simulink model "MATE_PMSMDynamicSwitches"  (R2024b)
settings: Solver=FixedStepDiscrete  StartTime=0.0  StopTime=0.6  RelTol=1e-3  AbsTol=1e-3
PostLoadFcn:
  | Ts = 2e-6;
  | PMSMDynamicSwitches_init
InitFcn:
  | Ts = 2e-6;
  | PMSMDynamicSwitches_init
values from neighbouring files (symbols this model uses):
  J = 0.2    [PMSMDynamicSwitches_init.m]
  Tmax = 1.5*N*PM*Imax    (= 27)    [PMSMDynamicSwitches_init.m]
  Tsc = 1/fc    (= 5e-05)    [PMSMDynamicSwitches_init.m]
libraries: fl_lib x24, nesl_utility x19, simulink x3, ee_lib x3, batteryecm_lib x1, eePmsmFieldOrientedControl x1
(part 1 of 2)
Description:
  | Three-Phase PMSM Drive
settings Model: DataTypeOverride=Off  ModifiedByFormat=KD  Creator=Kyle Diller  LastModifiedBy=KD
settings SolverCC: AutoScaleAbsTol=off  MaxConsecutiveMinStep=2  ZeroCrossAlgorithm=Adaptive  AlgebraicLoopSolver=TrustRegion  MaxZcPerStep=1
settings DataIOCC: LimitDataPoints=on  MaxDataPoints=690000  SaveFormat=Array  ReturnWorkspaceOutputs=off  SignalLoggingName=logsout_ee_pmsm_drive
settings OptimizationCC: BlockReduction=off  ConditionallyExecuteInputs=off  DefaultParameterBehavior=Inlined  InheritOutputTypeSmallerThanSingle=on  ReuseModelBlockBuffer=off  LifeSpan=inf
settings DebuggingCC: AlgebraicLoopMsg=error  MaxConsecutiveZCsMsg=none  IgnoredZcDiagnostic=none  SingleTaskRateTransMsg=error  UnconnectedInputMsg=warning  UnconnectedOutputMsg=warning  UnconnectedLineMsg=warning  AllowSymbolicDim=off  PregeneratedLibrarySubsystemCodeDiagnostic=none  SFUnexpectedBacktrackingDiag=warning  SFNoUnconditionalDefaultTransitionDiag=warning  SFExecutionAtInitializationDiag=none  ArithmeticOperatorsInVariantConditions=warning
settings HardwareCC: ProdBitPerPointer=32  ProdBitPerSizeT=32  ProdBitPerPtrDiffT=32  ProdLargestAtomicFloat=None  ProdIntDivRoundTo=Undefined  ProdEndianess=Unspecified  ProdWordSize=32  ProdHWDeviceType=ASIC/FPGA->ASIC/FPGA  TargetBitPerPointer=64  TargetBitPerSizeT=64  TargetBitPerPtrDiffT=64  TargetLongLongMode=on  TargetIntDivRoundTo=Zero  TargetEndianess=LittleEndian  TargetWordSize=64  TargetHWDeviceType=Custom Processor->MATLAB Host Computer  ProdEqTarget=off
settings ModelReferenceCC: EnableRefExpFcnMdlSchedulingChecks=on  PropagateSignalLabelsOutOfModel=off
settings SFSimCC: SimUseLocalCustomCode=off
settings RTWCC: RTWUseLocalCustomCode=off  GPUComputeCapability=3.5  DLArmComputeVersion=19.05
settings CodeAppCC: StateflowObjectComments=on
settings GRTTargetCC: TargetLangStandard=C89/C90 (ANSI)
settings ConfigComp: CovMetricSettings=dw  CovSaveCumulativeToWorkspaceVar=on  CovSaveSingleToWorkspaceVar=on  CovExternalEMLEnable=off  CovSFcnEnable=off
settings SimscapeCC: SimscapeLogType=all  SimscapeLogSimulationStatistics=on  SimscapeLogName=simlog_ee_pmsm_drive  SimscapeLogDataHistory=690000

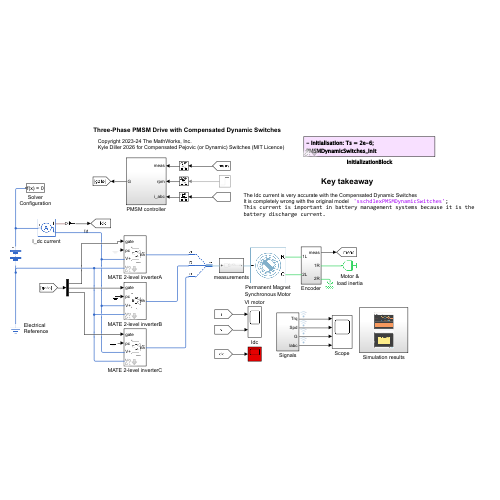
[thumbnail: Simulink's stored preview of the top-level diagram]
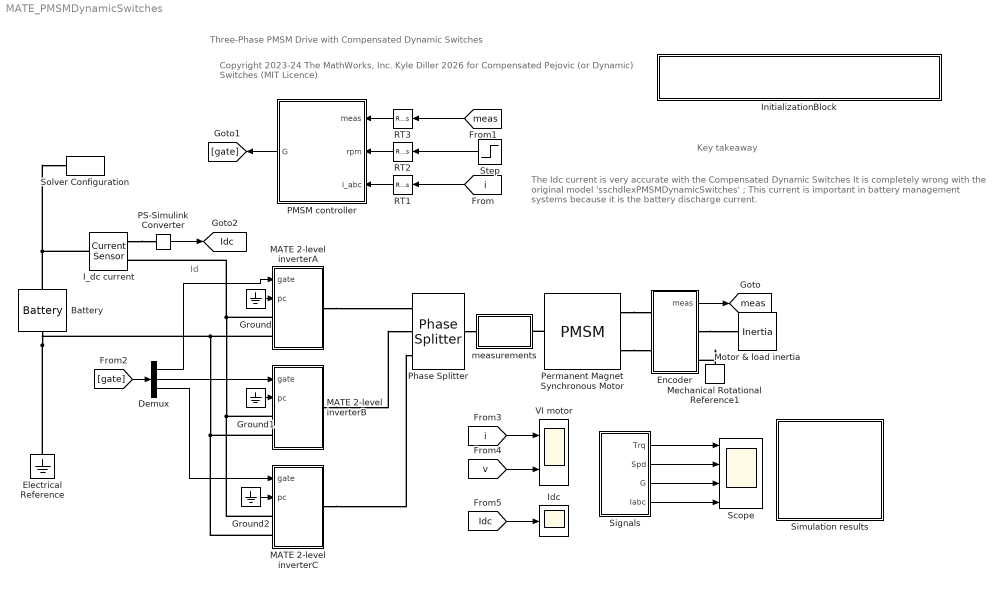
== system MATE_PMSMDynamicSwitches ==
  note: Key takeaway
  note: The Idc current is very accurate with the Compensated Dynamic Switches
      | It is completely wrong with the original model 'sschdlexPMSMDynamicSwitches' ;
      | This current is important in battery management systems because it is the battery discharge current.
  note: Id
  note: Three-Phase PMSM Drive with Compensated Dynamic Switches
  note: Copyright 2023-24 The MathWorks, Inc.
      | Kyle Diller 2026 for Compensated Pejovic (or Dynamic) Switches (MIT Licence)
  Battery : batteryecm_lib/Battery  Vnom=48 V  prm_dir=1  R1_dis=2 Ohm  R1_ch=2 Ohm  R1=0.001 Ohm  prm_AH=1  AH=14000 hr*A  V1=470 V  AH1=5000 hr*A  prm_R2=1  R2=inf Ohm  Tmeas=298.15 K  charge_measurement_port=simscape.enum.battery.enable.no  prm_dyn=1  Rp1=0.005 Ohm  tau1=30 s  Rp2=0.005 Ohm  tau2=30 s  Rp3=0.005 Ohm  tau3=30 s  Rp4=0.005 Ohm  tau4=30 s  Rp5=0.005 Ohm  tau5=30 s  prm_fade=1  N_fade=100  AH_fade=45 hr*A  R1_fade=2.02 Ohm  R1_ch_fade=2.02 Ohm  V1_fade=10.35 V  prm_age=1  prm_age_OCV=1  OCV_age=0.9  SOC_age=60  Tmeas_age=298.15 K  delta_time_age_vec=[0] d  temperature_age_vec=[273] K  OCV_scaling_age=2.2134e6  OCV_offset_age=1.632e6  temp_exp_age=0.515833569 V  t_exp_age=0.75  Vnom_T2=12 V  R1_T2=2.2 Ohm  R1_T2_dis=2.2 Ohm  R1_T2_ch=2.2 Ohm  V1_T2=11.4 V  R2_T2=2200 Ohm  Rp1_T2=0.005 Ohm  tau1_T2=30 s  Rp2_T2=0.005 Ohm  tau2_T2=30 s  Rp3_T2=0.005 Ohm  tau3_T2=30 s  Rp4_T2=0.005 Ohm  tau4_T2=30 s  Rp5_T2=0.005 Ohm  tau5_T2=30 s  Tmeas2=273.15 K  thermal_port=simscape.enum.thermaleffects.omit  thermal_mass=30000 J/K  i_specify=off  i_priority=None  i=0 A  i_nominal_specify=off  i_nominal_value=1  i_nominal_unit=A  v_specify=off  v_priority=None  v=0 V  v_nominal_specify=off  v_nominal_value=1  v_nominal_unit=V  charge_specify=on  charge_priority=High  charge=7000 hr*A  charge_nominal_specify=off  charge_nominal_value=1  charge_nominal_unit=A*hr  num_cycles_specify=off  num_cycles_priority=High  num_cycles=0  num_cycles_nominal_specify=off  num_cycles_nominal_value=1  num_cycles_nominal_unit=1  temperature_specify=off  temperature_priority=High  temperature=298.15 K  temperature_nominal_specify=off  temperature_nominal_value=1  temperature_nominal_unit=K
  Demux : Demux  Outputs=[2 2 2]
  Electrical Reference : fl_lib/Electrical/Electrical Elements/Electrical Reference
  Encoder : Subsystem
  Ground : Ground
  Ground1 : Ground
  Ground2 : Ground
  I_dc current : fl_lib/Electrical/Electrical Sensors/Current Sensor
  Idc : Scope
  InitializationBlock : Subsystem  AncestorBlock=simetranss/Usefulls/InitializationBlock  mask(Model Functions){InitVar=Ts = 2e-6;, InitFile=PMSMDynamicSwitches_init, prel=off, posl=on, inif=on}
      mask prompts: InitVar "Initialisation variables"; InitFile "Initialisation file (.m or .p)"; prel "Preload Function"; posl "PostLoad Function"; inif "InitFcn"
      mask init:
      | InitAll=[InitVar 10 InitFile];
      | if prel==1
      | 	set_param(bdroot, 'PreLoadFcn', InitAll);
      | else
      | 	set_param(bdroot, 'PreLoadFcn', '');
      | end
      | if inif==1
      | 	set_param(bdroot, 'InitFcn', InitAll);
      |     InitAll
      | else
      | 	set_param(bdroot, 'InitFcn', '');
      | end
      | 
      | if posl==1
      | 	set_param(bdroot, 'PostLoadFcn', InitAll);
      | else
      | 	set_param(bdroot, 'PostLoadFcn', '');
      | end
      | 
      | 
      | 
      | pos = get_param(gcb, 'Position');
      | width = pos(3) - pos(1); height = pos(4) - pos(2);
      mask DialogControl openfile Prompt: Open Initialisation file
      mask DialogControl openfile Callback:
      | ff1=get_param(gcb,'InitFile');
      | ff=replace(ff1,';','');
      | ff=replace(ff,'.m','');
      | ff=replace(ff,'.p','');
      | 
      | if ~isempty(strfind(ff1,'.p'))
      |     warning('p-file cannot be edited')
      | end
      | 
      | open(ff);
      mask Display:
      | text(5, height*0.5, [ ...
      |   ...
      | '- Initialisation: '  get_param(bdroot, 'InitFcn')  ...
      | ], ...
      | 'horizontalAlignment', 'left', 'verticalAlignment', 'middle') ;
  MATE 2-level inverterA : Subsystem  AncestorBlock=simetranss/FPGA/MATE 2-level inverter Pejovic  mask(MATE Compensated Pejovic 2-level inverter){Lon=1e-6, Ts=Ts}
      mask prompts: Lon "Conduction state inductance (H)"; Ts "Sample time (s)"
      mask help:
      | This block implements a 2-level IGBT/diode inverter with Pejovic switches.
      | The 2 switch are compensated at switching instant to transfer the L/C energy between the 2 switches, resulting in much better accuracy, much less spurious oscillation and power losses.
      |
      | The model supports dead-time on the gates. Internal logic makes the anti-parallel diode acts according to current direction when both gates are OFF.
      |
      | This model cannot interpolate or oversampled the gate action. Use of MATE 2-level inverter SWFHIZ is advised for this requirement.
      |
      | The 'pc' entry stands for 'precharge' when this input equals one and the upper gate level is one also, the upper switch acts as a simple resistance equal to the Pejovic resistance (L/h). In some converters, this property can be used to precharge the converter, as a pre-insersion resistance would do.
  MATE 2-level inverterB : Subsystem  AncestorBlock=simetranss/FPGA/MATE 2-level inverter Pejovic  mask(MATE Compensated Pejovic 2-level inverter){Lon=1e-6, Ts=Ts}
      mask prompts: Lon "Conduction state inductance (H)"; Ts "Sample time (s)"
      mask help:
      | This block implements a 2-level IGBT/diode inverter with Pejovic switches.
      | The 2 switch are compensated at switching instant to transfer the L/C energy between the 2 switches, resulting in much better accuracy, much less spurious oscillation and power losses.
      |
      | The model supports dead-time on the gates. Internal logic makes the anti-parallel diode acts according to current direction when both gates are OFF.
      |
      | This model cannot interpolate or oversampled the gate action. Use of MATE 2-level inverter SWFHIZ is advised for this requirement.
      |
      | The 'pc' entry stands for 'precharge' when this input equals one and the upper gate level is one also, the upper switch acts as a simple resistance equal to the Pejovic resistance (L/h). In some converters, this property can be used to precharge the converter, as a pre-insersion resistance would do.
  MATE 2-level inverterC : Subsystem  AncestorBlock=simetranss/FPGA/MATE 2-level inverter Pejovic  mask(MATE Compensated Pejovic 2-level inverter){Lon=1e-6, Ts=Ts}
      mask prompts: Lon "Conduction state inductance (H)"; Ts "Sample time (s)"
      mask help:
      | This block implements a 2-level IGBT/diode inverter with Pejovic switches.
      | The 2 switch are compensated at switching instant to transfer the L/C energy between the 2 switches, resulting in much better accuracy, much less spurious oscillation and power losses.
      |
      | The model supports dead-time on the gates. Internal logic makes the anti-parallel diode acts according to current direction when both gates are OFF.
      |
      | This model cannot interpolate or oversampled the gate action. Use of MATE 2-level inverter SWFHIZ is advised for this requirement.
      |
      | The 'pc' entry stands for 'precharge' when this input equals one and the upper gate level is one also, the upper switch acts as a simple resistance equal to the Pejovic resistance (L/h). In some converters, this property can be used to precharge the converter, as a pre-insersion resistance would do.
  Mechanical Rotational Reference1 : fl_lib/Mechanical/Rotational Elements/Mechanical Rotational Reference
  Motor & load inertia : fl_lib/Mechanical/Rotational Elements/Inertia  inertia=J kg*m^2  num_ports=foundation.enum.numPorts2.one  w_specify=on  w_priority=High  w=0 rpm  w_nominal_specify=off  w_nominal_value=1  w_nominal_unit=rad/s  t_specify=off  t_priority=High  t=0 N*m  t_nominal_specify=off  t_nominal_value=1  t_nominal_unit=N*m
  PMSM controller : Subsystem
  PS-Simulink Converter : nesl_utility/PS-Simulink Converter  PhysicalDomain=network_engine_domain  SubClassName=ps_output  LeftPortType=input  RightPortType=output  PseudoPeriodic=off  Frequencies=[]  VectorFormat=inherit  Unit=inherit  AffineConversion=off
  Permanent Magnet Synchronous Motor : ee_lib/Electromechanical/Permanent Magnet/PMSM  port_option=ee.enum.threePhasePort.composite  winding_type=ee.enum.statorconnection.wye  machine_param=ee.enum.pmsm.parameterization.constant  nPolePairs=N  pmflux_param=ee.enum.pmflux.fluxlinkage  pm_flux_linkage=PM Wb  torque_constant=0.18 N*m/A  back_emf_constant=0.18 V/(rad/s)  stator_param=ee.enum.statorparam.LdLqL0  Ld=Ld H  Lq=Lq H  idVec=[-200, 0, 200] A  iqVec=[-200, 0, 200] A  LdMatrix=0.0002 * ones(3, 3) H  LqMatrix=0.0002 * ones(3, 3) H  PmMatrix=0.1 * ones(3, 3) Wb  ktMatrix=0.18 * ones(3, 3) N*m/A  keMatrix=0.18 * ones(3, 3) V/(rad/s)  L0=L0 H  Ls=0.0002 H  Lm=0.00002 H  Ms=0.00002 H  Rs=Rs Ohm  zero_sequence=ee.enum.park.zerosequence.exclude  axes_param=ee.enum.rotorangle.qaxis  loss_param=ee.enum.ironloss.none  losses_oc=[0, 0, 0] W  losses_sc=[0, 0, 0] W  f_losses=60 Hz  Isc_losses=95 A  J=0 kg*m^2  lam=0 N*m/(rad/s)  i_d_specify=off  i_d_priority=None  i_d=0 A  i_d_nominal_specify=off  i_d_nominal_value=1  i_d_nominal_unit=A  i_q_specify=off  i_q_priority=None  i_q=0 A  i_q_nominal_specify=off  i_q_nominal_value=1  i_q_nominal_unit=A  torque_specify=off  torque_priority=None  torque=0 N*m  torque_nominal_specify=off  torque_nominal_value=1  torque_nominal_unit=N*m  angular_velocity_specify=on  angular_velocity_priority=None  angular_velocity=0 rpm  angular_velocity_nominal_specify=off  angular_velocity_nominal_value=1  angular_velocity_nominal_unit=rpm  angular_position_specify=on  angular_position_priority=High  angular_position=0 rad  angular_position_nominal_specify=off  angular_position_nominal_value=1  angular_position_nominal_unit=deg  alpha=3.93e-3 1/K  alpha_flux=-0.001 1/K  Tmeas=298.15 K  stator_thermal_mass=100 J/K  rotor_thermal_mass=200 J/K  Rm_percent_rotor=90  Rd_percent_rotor=30  temperatureA_specify=off  temperatureA_priority=High  temperatureA=25 degC  temperatureA_nominal_specify=off  temperatureA_nominal_value=1  temperatureA_nominal_unit=degC  temperatureB_specify=off  temperatureB_priority=High  temperatureB=25 degC  temperatureB_nominal_specify=off  temperatureB_nominal_value=1  temperatureB_nominal_unit=degC  temperatureC_specify=off  temperatureC_priority=High  temperatureC=25 degC  temperatureC_nominal_specify=off  temperatureC_nominal_value=1  temperatureC_nominal_unit=degC  temperatureR_specify=off  temperatureR_priority=High  temperatureR=25 degC  temperatureR_nominal_specify=off  temperatureR_nominal_value=1  temperatureR_nominal_unit=degC
      settings: InternalSimscapePortConfiguration="{\"Bottom\":[],\"Left\":[{\"id\":\"N\",\"label\":\"~\",\"type\":\"foundation.electrical.three_phase\"}],\"Right\":[{\"id\":\"R\",\"label\":\"R\",\"type\":\"foundation.mechanical.rotational.rotational\"},{\"id\":\"C\",\"label\":\"C\",\"type\":\"foundation.mechanical.rotational.rotational\"}],\"Top\":[]}"
  Phase Splitter : ee_lib/Connectors & References/Phase Splitter
  RT1 : RateTransition  OutPortSampleTime=Tsc
  RT2 : RateTransition  OutPortSampleTime=Tsc
  RT3 : RateTransition  OutPortSampleTime=Tsc
  Scope : Scope  NumInputPorts=4
  "Signals " : Subsystem
  Simulation results : Subsystem
  Solver Configuration : nesl_utility/Solver Configuration  PhysicalDomain=network_engine_domain  SubClassName=solver  LeftPortType=input  RightPortType=generic  Tones=[]  Harmonics=[]  SimulateNoise=off  Profile=off  UseLocalSampling=off  EnableSwitchedLinearOptims=on  FrequencyDomain=off  UseCCode=off  RelTol=0.001  AbsTol=1e-06  MinStep=1e-09  ToWorkspace=off  RevertToSquareIcSolve=off  NumHomotopyIterations=100  PhasorMode=off  PhasorModeNumHarmonics=1  ConsistencySolver=NEWTON_FTOL  IndexReductionMethod=DerivativeReplacement  DoDC=off  ResidualTolerance=1e-9  ConsistencyTolSource=GLOBAL  ConsistencyAbsTol=0.001  ConsistencyRelTol=0.001  ConsistencyTolFactor=0.001  UseLocalSolver=on  LocalSolverChoice=NE_PARTITIONING_ADVANCER  ResolveIndetEquations=on  FunctionEvalNumThread=1  LocalSolverSampleTime=Ts  DoFixedCost=on  MaxNonlinIter=4  MaxModeIter=2  ComputeImpulses=off  ImpulseIterations=2  LinearAlgebra=auto  LinearAlgebraNumThread=0  EquationFormulation=NE_TIME_EF  DelaysMemoryBudget=1024  AutomaticFiltering=on  FilteringTimeConstant=0.001  PartitionStorageMethod=AS_NEEDED  PartitionMemoryBudget=1024  PartitionMethod=FAST  MultibodyUseLocalSolver=off  MultibodyLocalSolverChoice=ODE1  MultibodyLocalSolverSampleTime=0.001
  Step : Step  Time=0.1  After=500  SampleTime=0
  VI motor : Scope  NumInputPorts=2
  measurements : Subsystem
  tag scope: Idc=global, meas=global
  wires:
  Step/1 -> RT2/1
  RT3/1 -> PMSM controller/1(meas)
  RT2/1 -> PMSM controller/2(rpm)
  RT1/1 -> PMSM controller/3(i_abc)
  "Signals "/2(Spd) -> Scope/2
  "Signals "/4(Iabc) -> Scope/4
  "Signals "/3(G) -> Scope/3
  "Signals "/1(Trq) -> Scope/1
  [i] -> RT1/1
  Encoder/1(meas) -> [meas]
  [meas] -> RT3/1
  PMSM controller/1(G) -> [gate]
  Demux/2 -> MATE 2-level inverterB/1(gate)
  Demux/1 -> MATE 2-level inverterA/1(gate)
  Demux/3 -> MATE 2-level inverterC/1(gate)
  [gate] -> Demux/1
  [i] -> VI motor/1
  [v] -> VI motor/2
  PS-Simulink Converter/1 -> [Idc]
  [Idc] -> Idc/1
  Ground/1 -> MATE 2-level inverterA/2(pc)
  Ground1/1 -> MATE 2-level inverterB/2(pc)
  Ground2/1 -> MATE 2-level inverterC/2(pc)
  connections:
  Battery/LConn1 -- I_dc current/LConn1 -- Solver Configuration/RConn1
  Permanent Magnet Synchronous Motor/RConn1 -- Encoder/LConn1
  Permanent Magnet Synchronous Motor/RConn2 -- Encoder/LConn2
  Encoder/RConn1 -- Motor & load inertia/LConn1
  Mechanical Rotational Reference1/LConn1 -- Encoder/RConn2
  Electrical Reference/LConn1 -- MATE 2-level inverterA/LConn2 -- MATE 2-level inverterC/LConn2 -- MATE 2-level inverterB/LConn2 -- Battery/RConn1
  I_dc current/RConn1 -- PS-Simulink Converter/LConn1
  MATE 2-level inverterA/LConn1 -- I_dc current/RConn2 -- MATE 2-level inverterC/LConn1 -- MATE 2-level inverterB/LConn1
  MATE 2-level inverterA/RConn1 -- Phase Splitter/RConn1
  MATE 2-level inverterB/RConn1 -- Phase Splitter/RConn2
  MATE 2-level inverterC/RConn1 -- Phase Splitter/RConn3
  Phase Splitter/LConn1 -- measurements/LConn1
  Permanent Magnet Synchronous Motor/LConn1 -- measurements/RConn1

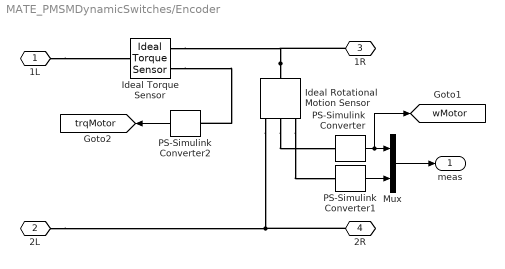
== system MATE_PMSMDynamicSwitches/Encoder ==
  Ideal Rotational Motion Sensor : fl_lib/Mechanical/Mechanical Sensors/Ideal Rotational Motion Sensor  reference=foundation.enum.MeasurementReference.difference  acceleration_port=false  velocity_port=true  position_port=true  wrap_angle=simscape.enum.onoff.off  offset=0 deg
  Ideal Torque Sensor : fl_lib/Mechanical/Mechanical Sensors/Ideal Torque Sensor
  Mux : Mux  Inputs=2
  PS-Simulink Converter : nesl_utility/PS-Simulink Converter  PhysicalDomain=network_engine_domain  SubClassName=ps_output  LeftPortType=input  RightPortType=output  PseudoPeriodic=off  Frequencies=[]  VectorFormat=1-D array  Unit=rad/s  AffineConversion=off
  PS-Simulink Converter1 : nesl_utility/PS-Simulink Converter  PhysicalDomain=network_engine_domain  SubClassName=ps_output  LeftPortType=input  RightPortType=output  PseudoPeriodic=off  Frequencies=[]  VectorFormat=1-D array  Unit=rad  AffineConversion=off
  PS-Simulink Converter2 : nesl_utility/PS-Simulink Converter  PhysicalDomain=network_engine_domain  SubClassName=ps_output  LeftPortType=input  RightPortType=output  PseudoPeriodic=off  Frequencies=[]  VectorFormat=1-D array  Unit=N*m  AffineConversion=off
  1L : PMIOPort  Side=Left
  2L : PMIOPort  Port=2  Side=Left
  1R : PMIOPort  Port=3  Side=Right
  2R : PMIOPort  Port=4  Side=Right
  meas : Outport  VectorParamsAs1DForOutWhenUnconnected=off
  tag scope: trqMotor=global, wMotor=global
  wires:
  PS-Simulink Converter2/1 -> [trqMotor]
  Mux/1 -> meas/1
  PS-Simulink Converter1/1 -> Mux/2
  PS-Simulink Converter/1 -> [wMotor], Mux/1
  connections:
  Ideal Torque Sensor/RConn2 -- PS-Simulink Converter2/LConn1
  1L/RConn1 -- Ideal Torque Sensor/LConn1
  2R/RConn1 -- 2L/RConn1 -- Ideal Rotational Motion Sensor/RConn1
  Ideal Rotational Motion Sensor/LConn1 -- 1R/RConn1 -- Ideal Torque Sensor/RConn1
  Ideal Rotational Motion Sensor/RConn2 -- PS-Simulink Converter/LConn1
  Ideal Rotational Motion Sensor/RConn3 -- PS-Simulink Converter1/LConn1

== system MATE_PMSMDynamicSwitches/InitializationBlock ==

== system MATE_PMSMDynamicSwitches/MATE 2-level inverterA ==
  gate : Inport
  pc : Inport  Port=2
  Add : Sum  Inputs=-+
  Demux2 : Demux  Outputs=2
  IGBT/Diode logic : Subsystem
  Unit Delay2 : UnitDelay  SampleTime=Ts  HasFrameUpgradeWarning=on
  lower : Subsystem  AncestorBlock=simetranss/FPGA/Pejovic L-C-switch component  mask(Pejovic Element for FPGA simulation){typ=2-level inverter switch, Lon=Lon, L=1, C=1, otherSW='coming soon', Ts=Ts, pcbp=off}
      mask prompts: typ "Element type"; Lon "Switch equivalent ON inductance (H)"; L "Inductor inductance (H)"; C "Capacitor capacitance (F)"; otherSW "Linked Compensated switch name"; Ts "Sample Time (s)"; pcbp "Precharge bypass (inverter only)"
      mask help:
      | Pejovic L-C-Switch element  in SimScape
      |
      | Implements either  an inductor, a capacitor or a switch using the Pejovic constant admittance method.
      |
      | For the Switch option, the user only has to select the equivalent ON-state inductance of the model, the corresponding Capacitance is computed internally. In the Pejovic model, Ts/Lon=Coff/Ts (Backward Euler) resulting in a constant admittance for the DAE solver.
      |
      |
      | Input signals;
      |
      | gate: the switch gate value (1 for ON , 0 for OFF) (with Switch option)
      mask init:
      | block=gcb;
      | Xcomp=0;
      | 
      | typp=get_param(block,'typ');
      | bp=get_param(block,'pcbp');
      | if isequal(typp,'Switch')
      |     replace_block (block ,'Followlinks' ,'on' ,'Name' ,'gate' ,'BlockType' ,'Constant' ,'Inport' ,'noprompt' ); 
      |     replace_block (block ,'Followlinks' ,'on' ,'Name' ,'init_in' ,'BlockType' ,'Inport' ,'Constant' ,'noprompt'  );
      |     replace_block (block ,'Followlinks' ,'on' ,'Name' ,'init_out' ,'BlockType' ,'Outport' ,'Terminator' ,'noprompt'  );
      |     Rsw=Lon/Ts;
      |     txt='Switch';
      | 
      | elseif isequal(typp,'Inductor')
      |     replace_block (block ,'Followlinks' ,'on' ,'Name' ,'gate' ,'BlockType' ,'Inport' ,'Constant' ,'noprompt' ); 
      |     set_param([block '/gate'],'Value','1');
      |     replace_block (block ,'Followlinks' ,'on' ,'Name' ,'init_in' ,'BlockType' ,'Inport' ,'Constant' ,'noprompt'  ); 
      |     replace_block (block ,'Followlinks' ,'on' ,'Name' ,'init_out' ,'BlockType' ,'Outport' ,'Terminator' ,'noprompt'  );
      |     Rsw=L/Ts;
      |     txt='L';
      | elseif isequal(typp,'Capacitor')
      |     replace_block (block ,'Followlinks' ,'on' ,'Name' ,'gate' ,'BlockType' ,'Inport' ,'Constant' ,'noprompt' ); 
      |     set_param([block '/gate'],'Value','0');
      |     replace_block (block ,'Followlinks' ,'on' ,'Name' ,'init_in' ,'BlockType' ,'Inport' ,'Constant' ,'noprompt'  );
      |     replace_block (block ,'Followlinks' ,'on' ,'Name' ,'init_out' ,'BlockType' ,'Outport' ,'Terminator' ,'noprompt'  );
      |     Rsw=Ts/C;
      |     txt='C';
      | elseif isequal(typp,'2-level inverter switch')
      |     replace_block (block ,'Followlinks' ,'on' ,'Name' ,'gate' ,'BlockType' ,'Constant' ,'Inport' ,'noprompt' ); 
      |     replace_block (block ,'Followlinks' ,'on' ,'Name' ,'init_in' ,'BlockType' ,'Constant' ,'Inport','noprompt'  );
      |     replace_block (block ,'Followlinks' ,'on' ,'Name' ,'init_out' ,'BlockType' ,'Terminator' ,'Outport' ,'noprompt'  );
      |     Rsw=Lon/Ts;
      |     txt='Inverter half';
      |     Xcomp=1;
      | 
      | else
      | end
      | 
      | if isequal(typp,'2-level inverter switch')  && isequal(bp,'on')
      |         replace_block (block ,'Followlinks' ,'on' ,'Name' ,'Bypass' ,'BlockType' ,'Ground' ,'Inport' ,'noprompt' ); 
      | else
      |         replace_block (block ,'Followlinks' ,'on' ,'Name' ,'Bypass' ,'BlockType' ,'Inport' ,'Ground' ,'noprompt' ); 
      | end
      | 
      | 
      | 
      | 
      | if Ts>2e-6
      |     %warndlg(['Sample Time of ' num2str(Ts) ' s. may be somehow large for the Pejovic switch to be accurate. Sample time below 2 us are recommended.'])
      | end
      mask TypeOptions typ: Switch | Inductor | Capacitor | 2-level inverter switch
      mask Display: disp(txt)
  upper : Subsystem  AncestorBlock=simetranss/FPGA/Pejovic L-C-switch component  mask(Pejovic Element for FPGA simulation){typ=2-level inverter switch, Lon=Lon, L=1, C=1, otherSW='coming soon', Ts=Ts, pcbp=on}
      mask prompts: typ "Element type"; Lon "Switch equivalent ON inductance (H)"; L "Inductor inductance (H)"; C "Capacitor capacitance (F)"; otherSW "Linked Compensated switch name"; Ts "Sample Time (s)"; pcbp "Precharge bypass (inverter only)"
      mask help:
      | Pejovic L-C-Switch element  in SimScape
      |
      | Implements either  an inductor, a capacitor or a switch using the Pejovic constant admittance method.
      |
      | For the Switch option, the user only has to select the equivalent ON-state inductance of the model, the corresponding Capacitance is computed internally. In the Pejovic model, Ts/Lon=Coff/Ts (Backward Euler) resulting in a constant admittance for the DAE solver.
      |
      |
      | Input signals;
      |
      | gate: the switch gate value (1 for ON , 0 for OFF) (with Switch option)
      mask init: same as MATE_PMSMDynamicSwitches/MATE 2-level inverterA/lower
      mask TypeOptions typ: Switch | Inductor | Capacitor | 2-level inverter switch
      mask Display: disp(txt)
  V+ : PMIOPort  Side=Left
  Va : PMIOPort  Port=2  Side=Right
  V- : PMIOPort  Port=3  Side=Left
  wires:
  pc/1 -> upper/3(Bypass)
  lower/1(init_out) -> upper/2(init_in)
  upper/1(init_out) -> lower/2(init_in)
  Demux2/1 -> upper/1(gate)
  Demux2/2 -> lower/1(gate)
  [iout] -> IGBT/Diode logic/2(u)
  gate/1 -> IGBT/Diode logic/1(In1)
  IGBT/Diode logic/1(UpperLower) -> Demux2/1
  Add/1 -> Unit Delay2/1
  Unit Delay2/1 -> [iout]
  upper/2(iout) -> Add/1
  lower/2(iout) -> Add/2
  connections:
  lower/RConn1 -- V-/RConn1
  upper/LConn1 -- V+/RConn1
  lower/LConn1 -- Va/RConn1 -- upper/RConn1

== system MATE_PMSMDynamicSwitches/MATE 2-level inverterB ==
  gate : Inport
  pc : Inport  Port=2
  Add : Sum  Inputs=-+
  Demux2 : Demux  Outputs=2
  IGBT/Diode logic : Subsystem
  Unit Delay2 : UnitDelay  SampleTime=Ts  HasFrameUpgradeWarning=on
  lower : Subsystem  AncestorBlock=simetranss/FPGA/Pejovic L-C-switch component  mask(Pejovic Element for FPGA simulation){typ=2-level inverter switch, Lon=Lon, L=1, C=1, otherSW='coming soon', Ts=Ts, pcbp=off}
      mask prompts: typ "Element type"; Lon "Switch equivalent ON inductance (H)"; L "Inductor inductance (H)"; C "Capacitor capacitance (F)"; otherSW "Linked Compensated switch name"; Ts "Sample Time (s)"; pcbp "Precharge bypass (inverter only)"
      mask help:
      | Pejovic L-C-Switch element  in SimScape
      |
      | Implements either  an inductor, a capacitor or a switch using the Pejovic constant admittance method.
      |
      | For the Switch option, the user only has to select the equivalent ON-state inductance of the model, the corresponding Capacitance is computed internally. In the Pejovic model, Ts/Lon=Coff/Ts (Backward Euler) resulting in a constant admittance for the DAE solver.
      |
      |
      | Input signals;
      |
      | gate: the switch gate value (1 for ON , 0 for OFF) (with Switch option)
      mask init: same as MATE_PMSMDynamicSwitches/MATE 2-level inverterA/lower
      mask TypeOptions typ: Switch | Inductor | Capacitor | 2-level inverter switch
      mask Display: disp(txt)
  upper : Subsystem  AncestorBlock=simetranss/FPGA/Pejovic L-C-switch component  mask(Pejovic Element for FPGA simulation){typ=2-level inverter switch, Lon=Lon, L=1, C=1, otherSW='coming soon', Ts=Ts, pcbp=on}
      mask prompts: typ "Element type"; Lon "Switch equivalent ON inductance (H)"; L "Inductor inductance (H)"; C "Capacitor capacitance (F)"; otherSW "Linked Compensated switch name"; Ts "Sample Time (s)"; pcbp "Precharge bypass (inverter only)"
      mask help:
      | Pejovic L-C-Switch element  in SimScape
      |
      | Implements either  an inductor, a capacitor or a switch using the Pejovic constant admittance method.
      |
      | For the Switch option, the user only has to select the equivalent ON-state inductance of the model, the corresponding Capacitance is computed internally. In the Pejovic model, Ts/Lon=Coff/Ts (Backward Euler) resulting in a constant admittance for the DAE solver.
      |
      |
      | Input signals;
      |
      | gate: the switch gate value (1 for ON , 0 for OFF) (with Switch option)
      mask init: same as MATE_PMSMDynamicSwitches/MATE 2-level inverterA/lower
      mask TypeOptions typ: Switch | Inductor | Capacitor | 2-level inverter switch
      mask Display: disp(txt)
  V+ : PMIOPort  Side=Left
  Va : PMIOPort  Port=2  Side=Right
  V- : PMIOPort  Port=3  Side=Left
  wires:
  pc/1 -> upper/3(Bypass)
  lower/1(init_out) -> upper/2(init_in)
  upper/1(init_out) -> lower/2(init_in)
  Demux2/1 -> upper/1(gate)
  Demux2/2 -> lower/1(gate)
  [iout] -> IGBT/Diode logic/2(u)
  gate/1 -> IGBT/Diode logic/1(In1)
  IGBT/Diode logic/1(UpperLower) -> Demux2/1
  Add/1 -> Unit Delay2/1
  Unit Delay2/1 -> [iout]
  upper/2(iout) -> Add/1
  lower/2(iout) -> Add/2
  connections:
  lower/RConn1 -- V-/RConn1
  upper/LConn1 -- V+/RConn1
  lower/LConn1 -- Va/RConn1 -- upper/RConn1

== system MATE_PMSMDynamicSwitches/MATE 2-level inverterC ==
  gate : Inport
  pc : Inport  Port=2
  Add : Sum  Inputs=-+
  Demux2 : Demux  Outputs=2
  IGBT/Diode logic : Subsystem
  Unit Delay2 : UnitDelay  SampleTime=Ts  HasFrameUpgradeWarning=on
  lower : Subsystem  AncestorBlock=simetranss/FPGA/Pejovic L-C-switch component  mask(Pejovic Element for FPGA simulation){typ=2-level inverter switch, Lon=Lon, L=1, C=1, otherSW='coming soon', Ts=Ts, pcbp=off}
      mask prompts: typ "Element type"; Lon "Switch equivalent ON inductance (H)"; L "Inductor inductance (H)"; C "Capacitor capacitance (F)"; otherSW "Linked Compensated switch name"; Ts "Sample Time (s)"; pcbp "Precharge bypass (inverter only)"
      mask help:
      | Pejovic L-C-Switch element  in SimScape
      |
      | Implements either  an inductor, a capacitor or a switch using the Pejovic constant admittance method.
      |
      | For the Switch option, the user only has to select the equivalent ON-state inductance of the model, the corresponding Capacitance is computed internally. In the Pejovic model, Ts/Lon=Coff/Ts (Backward Euler) resulting in a constant admittance for the DAE solver.
      |
      |
      | Input signals;
      |
      | gate: the switch gate value (1 for ON , 0 for OFF) (with Switch option)
      mask init: same as MATE_PMSMDynamicSwitches/MATE 2-level inverterA/lower
      mask TypeOptions typ: Switch | Inductor | Capacitor | 2-level inverter switch
      mask Display: disp(txt)
  upper : Subsystem  AncestorBlock=simetranss/FPGA/Pejovic L-C-switch component  mask(Pejovic Element for FPGA simulation){typ=2-level inverter switch, Lon=Lon, L=1, C=1, otherSW='coming soon', Ts=Ts, pcbp=on}
      mask prompts: typ "Element type"; Lon "Switch equivalent ON inductance (H)"; L "Inductor inductance (H)"; C "Capacitor capacitance (F)"; otherSW "Linked Compensated switch name"; Ts "Sample Time (s)"; pcbp "Precharge bypass (inverter only)"
      mask help:
      | Pejovic L-C-Switch element  in SimScape
      |
      | Implements either  an inductor, a capacitor or a switch using the Pejovic constant admittance method.
      |
      | For the Switch option, the user only has to select the equivalent ON-state inductance of the model, the corresponding Capacitance is computed internally. In the Pejovic model, Ts/Lon=Coff/Ts (Backward Euler) resulting in a constant admittance for the DAE solver.
      |
      |
      | Input signals;
      |
      | gate: the switch gate value (1 for ON , 0 for OFF) (with Switch option)
      mask init: same as MATE_PMSMDynamicSwitches/MATE 2-level inverterA/lower
      mask TypeOptions typ: Switch | Inductor | Capacitor | 2-level inverter switch
      mask Display: disp(txt)
  V+ : PMIOPort  Side=Left
  Va : PMIOPort  Port=2  Side=Right
  V- : PMIOPort  Port=3  Side=Left
  wires:
  pc/1 -> upper/3(Bypass)
  lower/1(init_out) -> upper/2(init_in)
  upper/1(init_out) -> lower/2(init_in)
  Demux2/1 -> upper/1(gate)
  Demux2/2 -> lower/1(gate)
  [iout] -> IGBT/Diode logic/2(u)
  gate/1 -> IGBT/Diode logic/1(In1)
  IGBT/Diode logic/1(UpperLower) -> Demux2/1
  Add/1 -> Unit Delay2/1
  Unit Delay2/1 -> [iout]
  upper/2(iout) -> Add/1
  lower/2(iout) -> Add/2
  connections:
  lower/RConn1 -- V-/RConn1
  upper/LConn1 -- V+/RConn1
  lower/LConn1 -- Va/RConn1 -- upper/RConn1

== system MATE_PMSMDynamicSwitches/PMSM controller ==
  meas : Inport
  rpm : Inport  Port=2
  i_abc : Inport  Port=3
  Bus Selector : BusSelector  OutputSignals=iabc [A],Reference,TqRef [N*m]
  Demux1 : Demux  Outputs=2
  PMSM Field-Oriented Control : eePmsmFieldOrientedControl/PMSM Field-Oriented Control  winding_type=Wye-wound  CtrlMode=Velocity control  Vnom=48  Pmax=Pmax  Tmax=Tmax*1.5  p=N  Vdc_on=10  Ts=Ts  Tsc=Tsc  CtrlType=PI control  Kp_w=60  Ki_w=300*2  Kv_w=1  Kaw_w=1000  RefType=Zero d-axis control  rpmVec=[0, 3000]  TqVec=[-100, 0, 100]  VdcVec=[300, 350]  PWMMode=SPWM: sinusoidal PWM  ModFactor=1  idMatrix=zeros(2,3,2)  iqMatrix=zeros(2,3,2)  psim=PM  Ld=0.00024  Lq=0.00029  Rs=0.01  AxisAlignment=Q-axis  Kp_id=0.1  Ki_id=10  Kaw_id=1000  Kp_iq=0.1  Ki_iq=10  Kaw_iq=1000  AxisPrio=Q-axis  ActZC=off  ActFF=on  ParamTypeFF=Constant parameters  LdFF=Ld  LqFF=Lq  psimFF=PM  idVect=[-200, 0, 200]  iqVect=[-200, 0, 200]  LdMatrix=0.0002 * ones(3, 3)  LqMatrix=0.0002 * ones(3, 3)  psimMatrix=0.04 * ones(3, 3)  CPWMMode=SPWM: sinusoidal PWM  fsw=fsw
  Rate Limiter : RateLimiter  RisingSlewLimit=Tmax/J  FallingSlewLimit=-Tmax/J  SampleTimeMode=inherited
  Vdc : Constant  Value=48  SampleTime=Tsc
  "rpm -> rad/s [mech.]" : Gain  Gain=2*pi/60
  G : Outport  VectorParamsAs1DForOutWhenUnconnected=off
  tag scope: iMotor=global, trqDemand=global, wDemand=global
  wires:
  PMSM Field-Oriented Control/1 -> G/1
  Vdc/1 -> PMSM Field-Oriented Control/5
  PMSM Field-Oriented Control/2 -> Bus Selector/1
  i_abc/1 -> PMSM Field-Oriented Control/2
  meas/1 -> Demux1/1
  Demux1/1 -> PMSM Field-Oriented Control/3
  Demux1/2 -> PMSM Field-Oriented Control/4
  Bus Selector/1 -> [iMotor]  "<iabc [A]>"
  Bus Selector/2 -> [wDemand]  "<Reference>"
  Bus Selector/3 -> [trqDemand]  "<TqRef [N*m]>"
  rpm/1 -> "rpm -> rad/s [mech.]"/1
  Rate Limiter/1 -> PMSM Field-Oriented Control/1
  "rpm -> rad/s [mech.]"/1 -> Rate Limiter/1

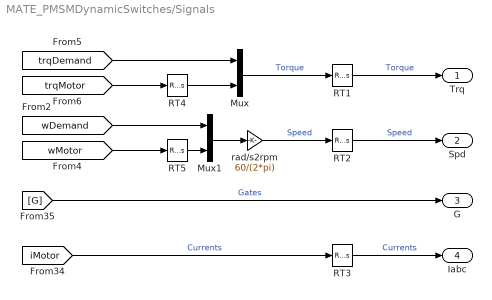
== system MATE_PMSMDynamicSwitches/Signals  ==
  Mux : Mux  Inputs=2
  Mux1 : Mux  Inputs=2
  RT1 : RateTransition  OutPortSampleTime=Ts
  RT2 : RateTransition  OutPortSampleTime=Ts
  RT3 : RateTransition  OutPortSampleTime=Ts
  RT4 : RateTransition  OutPortSampleTime=Tsc
  RT5 : RateTransition  OutPortSampleTime=Tsc
  rad/s2rpm : Gain  Gain=60/(2*pi)
  Trq : Outport  VectorParamsAs1DForOutWhenUnconnected=off
  Spd : Outport  Port=2  VectorParamsAs1DForOutWhenUnconnected=off
  G : Outport  Port=3  VectorParamsAs1DForOutWhenUnconnected=off
  Iabc : Outport  Port=4  VectorParamsAs1DForOutWhenUnconnected=off
  wires:
  [trqDemand] -> Mux/1
  [G] -> G/1  "Gates"
  Mux1/1 -> rad/s2rpm/1
  Mux/1 -> RT1/1  "Torque"
  [iMotor] -> RT3/1  "Currents"
  [wDemand] -> Mux1/1
  rad/s2rpm/1 -> RT2/1  "Speed"
  [trqMotor] -> RT4/1
  [wMotor] -> RT5/1
  RT1/1 -> Trq/1  "Torque"
  RT2/1 -> Spd/1  "Speed"
  RT3/1 -> Iabc/1  "Currents"
  RT4/1 -> Mux/2
  RT5/1 -> Mux1/2

== system MATE_PMSMDynamicSwitches/Simulation results ==
  note: df
  note: f g

== system MATE_PMSMDynamicSwitches/measurements ==
  Current and Voltage Sensor (Three-Phase) : ee_lib/Sensors & Transducers/Current and Voltage Sensor (Three-Phase)  vMeasurementType=ee.enum.vmeasurement.lg  outputUnit=ee.enum.unit.si  SRated=100e6 A*V  VRated=24e3 V  I_specify=off  I_priority=None  I=[0, 0, 0] A  I_nominal_specify=off  I_nominal_value=1  I_nominal_unit=A  V_specify=off  V_priority=None  V=[0, 0, 0] V  V_nominal_specify=off  V_nominal_value=1  V_nominal_unit=V
      settings: InternalSimscapePortConfiguration="{\"Bottom\":[],\"Left\":[{\"id\":\"N1\",\"label\":\"~1\",\"type\":\"foundation.electrical.three_phase\"}],\"Right\":[{\"id\":\"V_output\",\"label\":\"V\",\"type\":\"output\"},{\"id\":\"I_output\",\"label\":\"I\",\"type\":\"output\"},{\"id\":\"N2\",\"label\":\"~2\",\"type\":\"foundation.electrical.three_phase\"}],\"Top\":[]}"
  PS-Simulink Converter : nesl_utility/PS-Simulink Converter  PhysicalDomain=network_engine_domain  SubClassName=ps_output  LeftPortType=input  RightPortType=output  PseudoPeriodic=off  Frequencies=[]  VectorFormat=1-D array  Unit=A  AffineConversion=off
  PS-Simulink Converter1 : nesl_utility/PS-Simulink Converter  PhysicalDomain=network_engine_domain  SubClassName=ps_output  LeftPortType=input  RightPortType=output  PseudoPeriodic=off  Frequencies=[]  VectorFormat=inherit  Unit=inherit  AffineConversion=off
  + : PMIOPort  Side=Left
  - : PMIOPort  Port=2  Side=Right
  tag scope: i=global, v=global
  wires:
  PS-Simulink Converter1/1 -> [v]
  PS-Simulink Converter/1 -> [i]
  connections:
  PS-Simulink Converter1/LConn1 -- Current and Voltage Sensor (Three-Phase)/RConn1
  +/RConn1 -- Current and Voltage Sensor (Three-Phase)/LConn1
  -/RConn1 -- Current and Voltage Sensor (Three-Phase)/RConn3
  Current and Voltage Sensor (Three-Phase)/RConn2 -- PS-Simulink Converter/LConn1

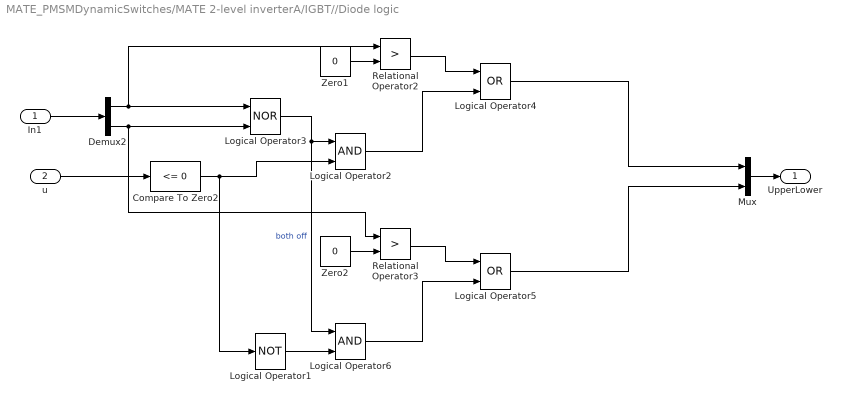
== system MATE_PMSMDynamicSwitches/MATE 2-level inverterA/IGBT//Diode logic ==
  In1 : Inport
  u : Inport  Port=2
  Compare To Zero2 : simulink/Logic and Bit Operations/Compare To Zero  relop=<=  OutDataTypeStr=uint8
  Demux2 : Demux  Outputs=2
  Logical Operator1 : Logic  Operator=NOT  AllPortsSameDT=off  OutDataTypeStr=boolean
  Logical Operator2 : Logic  AllPortsSameDT=off  OutDataTypeStr=boolean
  Logical Operator3 : Logic  Operator=NOR  AllPortsSameDT=off  OutDataTypeStr=boolean
  Logical Operator4 : Logic  Operator=OR  AllPortsSameDT=off  OutDataTypeStr=boolean
  Logical Operator5 : Logic  Operator=OR  AllPortsSameDT=off  OutDataTypeStr=boolean
  Logical Operator6 : Logic  AllPortsSameDT=off  OutDataTypeStr=boolean
  Mux : Mux  Inputs=2
  Relational Operator2 : RelationalOperator  Operator=>  OutDataTypeStr=boolean  InputSameDT=off
  Relational Operator3 : RelationalOperator  Operator=>  OutDataTypeStr=boolean  InputSameDT=off
  Zero1 : Constant  Value=0  OutDataTypeStr=Inherit: Inherit via back propagation
  Zero2 : Constant  Value=0  OutDataTypeStr=Inherit: Inherit via back propagation
  UpperLower : Outport
  wires:
  Mux/1 -> UpperLower/1
  Logical Operator5/1 -> Mux/2
  Logical Operator4/1 -> Mux/1
  In1/1 -> Demux2/1
  u/1 -> Compare To Zero2/1
  Logical Operator1/1 -> Logical Operator6/2
  Relational Operator3/1 -> Logical Operator5/1
  Logical Operator2/1 -> Logical Operator4/2
  Zero2/1 -> Relational Operator3/2
  Demux2/2 -> Relational Operator3/1, Logical Operator3/2
  Logical Operator6/1 -> Logical Operator5/2
  Compare To Zero2/1 -> Logical Operator2/2, Logical Operator1/1
  Zero1/1 -> Relational Operator2/2
  Logical Operator3/1 -> Logical Operator2/1, Logical Operator6/1  "both off"
  Relational Operator2/1 -> Logical Operator4/1
  Demux2/1 -> Relational Operator2/1, Logical Operator3/1

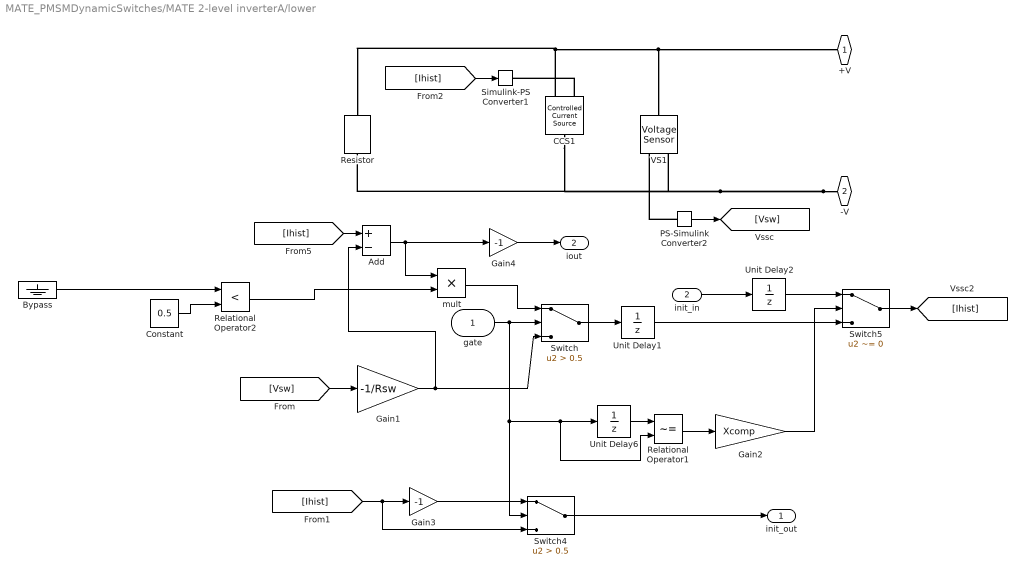
== system MATE_PMSMDynamicSwitches/MATE 2-level inverterA/lower ==
  gate : Inport
  init_in : Inport  Port=2
  Add : Sum  Inputs=+-
  Bypass : Ground
  CCS1 : fl_lib/Electrical/Electrical Sources/Controlled Current Source
  Constant : Constant  Value=0.5
  Gain1 : Gain  Gain=-1/Rsw
  Gain2 : Gain  Gain=Xcomp
  Gain3 : Gain  Gain=-1
  Gain4 : Gain  Gain=-1
  PS-Simulink Converter2 : nesl_utility/PS-Simulink Converter  PhysicalDomain=network_engine_domain  SubClassName=ps_output  LeftPortType=input  RightPortType=output  PseudoPeriodic=off  Frequencies=[]  VectorFormat=inherit  Unit=inherit  AffineConversion=off
  Relational Operator1 : RelationalOperator  Operator=~=  OutDataTypeStr=boolean  RndMeth=Simplest  InputSameDT=off
  Relational Operator2 : RelationalOperator  Operator=<  OutDataTypeStr=boolean  RndMeth=Simplest  InputSameDT=off
  Resistor : fl_lib/Electrical/Electrical Elements/Resistor  R=Rsw Ohm  i_specify=off  i_priority=None  i=0 A  i_nominal_specify=off  i_nominal_value=1  i_nominal_unit=A  v_specify=off  v_priority=None  v=0 V  v_nominal_specify=off  v_nominal_value=1  v_nominal_unit=V
  Simulink-PS Converter1 : nesl_utility/Simulink-PS Converter  PhysicalDomain=network_engine_domain  SubClassName=ps_input  LeftPortType=input  RightPortType=output  PseudoPeriodic=off  Frequencies=[]  NoiseDistribution=none  NoiseParameters=[]  Unit=1  AffineConversion=off  FilteringAndDerivatives=provide  SimscapeFilterOrder=1  InputFilterTimeConstant=0.001  UdotUserProvided=0
  Switch : Switch  Criteria=u2 > Threshold  Threshold=0.5  SaturateOnIntegerOverflow=off  InputSameDT=off
  Switch4 : Switch  Criteria=u2 > Threshold  Threshold=0.5  SaturateOnIntegerOverflow=off  InputSameDT=off
  Switch5 : Switch  Criteria=u2 ~= 0  Threshold=0.5  SaturateOnIntegerOverflow=off  InputSameDT=off
  Unit Delay1 : UnitDelay  SampleTime=-1  HasFrameUpgradeWarning=on
  Unit Delay2 : UnitDelay  SampleTime=Ts  HasFrameUpgradeWarning=on
  Unit Delay6 : UnitDelay  SampleTime=Ts  HasFrameUpgradeWarning=on
  VS1 : fl_lib/Electrical/Electrical Sensors/Voltage Sensor
  mult : Product
  +V : PMIOPort  Side=Left
  -V : PMIOPort  Port=2  Side=Right
  init_out : Outport
  iout : Outport  Port=2
  wires:
  Constant/1 -> Relational Operator2/2
  Unit Delay2/1 -> Switch5/1
  [Ihist] -> Gain3/1, Switch4/3
  Relational Operator2/1 -> mult/2
  Bypass/1 -> Relational Operator2/1
  mult/1 -> Switch/1
  [Ihist] -> Simulink-PS Converter1/1
  Switch/1 -> Unit Delay1/1
  [Vsw] -> Gain1/1
  PS-Simulink Converter2/1 -> [Vsw]
  [Ihist] -> Add/1
  Gain1/1 -> Switch/3, Add/2
  Add/1 -> Gain4/1, mult/1
  Unit Delay1/1 -> Switch5/3
  Switch4/1 -> init_out/1
  Gain3/1 -> Switch4/1
  Gain2/1 -> Switch5/2
  Unit Delay6/1 -> Relational Operator1/1
  gate/1 -> Switch4/2, Unit Delay6/1, Relational Operator1/2, Switch/2
  Relational Operator1/1 -> Gain2/1
  init_in/1 -> Unit Delay2/1
  Switch5/1 -> [Ihist]
  Gain4/1 -> iout/1
  connections:
  CCS1/RConn2 -- +V/RConn1 -- VS1/LConn1 -- Resistor/LConn1
  CCS1/RConn1 -- Simulink-PS Converter1/RConn1
  PS-Simulink Converter2/LConn1 -- VS1/RConn1
  -V/RConn1 -- VS1/RConn2 -- CCS1/LConn1 -- Resistor/RConn1
